simulink model "bh_explore_evassive_manoeuvre_automate"  (R2017b)
settings: Solver=ode45  StartTime=0.0  StopTime=20  FixedStep=0.001  RelTol=1e-5
undefined symbols (not defined in the file or in its folder): Peak_deg, Tw, vel_mpersec
libraries: simulink_extras x12, bh_cv_car_drc_library x1
settings Model: Creator=bhorton  LastModifiedBy=bhorton
settings SolverCC: ZeroCrossControl=EnableAll  ZeroCrossAlgorithm=Adaptive
settings DebuggingCC: SignalInfNanChecking=warning
settings ModelReferenceCC: ModelReferenceMinAlgLoopOccurrences=on

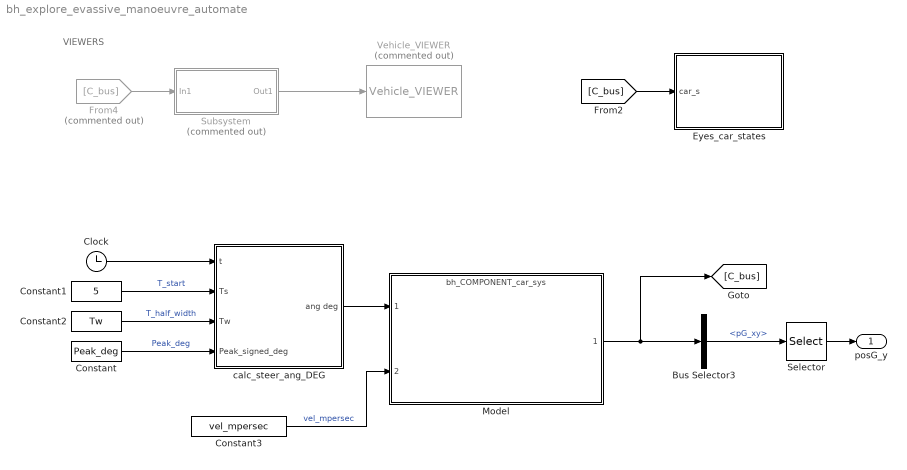
== system bh_explore_evassive_manoeuvre_automate ==
  note: VIEWERS
  Bus Selector3 : BusSelector  OutputSignals=states_G.pG_xy
  Clock : Clock
  Constant : Constant  Value=Peak_deg
  Constant1 : Constant  Value=5
  Constant2 : Constant  Value=Tw
  Constant3 : Constant  Value=vel_mpersec
  Eyes_car_states : Subsystem
  From4 : From  Commented=on  GotoTag=C_bus
  Model : ModelReference  ModelNameDialog=bh_COMPONENT_car_sys  SimulationMode=Normal  ModelReferenceVersion=1.261
  Selector : Selector  InputPortWidth=2  IndexOptions=Index vector (dialog)  Indices=2  OutputSizes=1
  Subsystem : Subsystem  Commented=on
  Vehicle_VIEWER : bh_cv_car_drc_library/CAR_things/Vehicle_VIEWER  Commented=on  wp_mat=[-1, -1; 2,2]  veh_ID_num=1  veh_init_xytheta=[0,0,0]  Ts=0.1
  calc_steer_ang_DEG : Subsystem
      mask Display: image(imread('evassive_PIC_01.JPG'))
  posG_y : Outport
  wires:
  [C_bus] -> Eyes_car_states/1(car_s)
  From4/1 -> Subsystem/1(In1)
  Subsystem/1(Out1) -> Vehicle_VIEWER/1
  Clock/1 -> calc_steer_ang_DEG/1(t)
  Constant/1 -> calc_steer_ang_DEG/4(Peak_signed_deg)  "Peak_deg"
  Constant1/1 -> calc_steer_ang_DEG/2(Ts)  "T_start"
  Constant2/1 -> calc_steer_ang_DEG/3(Tw)  "T_half_width"
  calc_steer_ang_DEG/1(ang deg) -> Model/1
  Constant3/1 -> Model/2  "vel_mpersec"
  Model/1 -> Bus Selector3/1, [C_bus]
  Bus Selector3/1 -> Selector/1  "<pG_xy>"
  Selector/1 -> posG_y/1

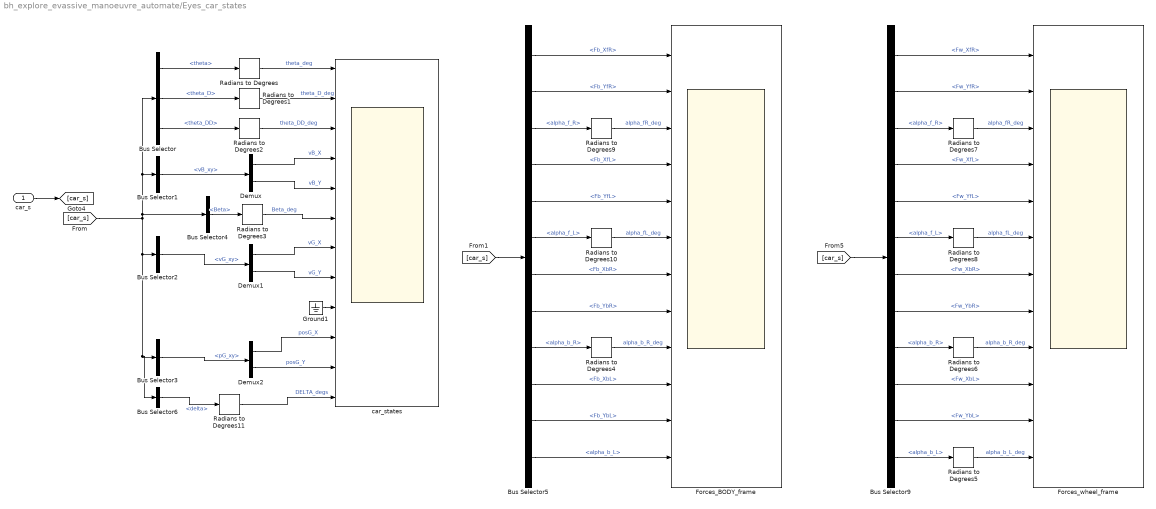
== system bh_explore_evassive_manoeuvre_automate/Eyes_car_states ==
  car_s : Inport
  Bus Selector : BusSelector  OutputSignals=states_B.theta,states_B.theta_D,states_B.theta_DD
  Bus Selector1 : BusSelector  OutputSignals=states_B.vB_xy
  Bus Selector2 : BusSelector  OutputSignals=states_G.vG_xy
  Bus Selector3 : BusSelector  OutputSignals=states_G.pG_xy
  Bus Selector4 : BusSelector  OutputSignals=states_B.Beta
  Bus Selector5 : BusSelector  OutputSignals=Force_BODY_frame.Fb_XfR,Force_BODY_frame.Fb_YfR,alpha.alpha_f_R,Force_BODY_frame.Fb_XfL,Force_BODY_frame.Fb_YfL,alpha.alpha_f_L,Force_BODY_frame.Fb_XbR,Force_BODY_frame.Fb_YbR,alpha.alpha_b_R,Force_BODY_frame.Fb_XbL,Force_BODY_frame.Fb_YbL,alpha.alpha_b_L
  Bus Selector6 : BusSelector  OutputSignals=wheel.delta
  Bus Selector9 : BusSelector  OutputSignals=Force_wheel_frame.Fw_XfR,Force_wheel_frame.Fw_YfR,alpha.alpha_f_R,Force_wheel_frame.Fw_XfL,Force_wheel_frame.Fw_YfL,alpha.alpha_f_L,Force_wheel_frame.Fw_XbR,Force_wheel_frame.Fw_YbR,alpha.alpha_b_R,Force_wheel_frame.Fw_XbL,Force_wheel_frame.Fw_YbL,alpha.alpha_b_L
  Demux : Demux  Outputs=2
  Demux1 : Demux  Outputs=2
  Demux2 : Demux  Outputs=2
  Forces_BODY_frame : Scope  NumInputPorts=12
  Forces_wheel_frame : Scope  NumInputPorts=12
  Ground1 : Ground
  Radians to Degrees{,1..11} (12 alike) : simulink_extras/Transformations/Radians to Degrees
  car_states : Scope  NumInputPorts=12
  wires:
  car_s/1 -> [car_s]
  [car_s] -> Bus Selector4/1, Bus Selector/1, Bus Selector1/1, Bus Selector6/1, Bus Selector3/1, Bus Selector2/1
  Bus Selector/1 -> Radians to Degrees/1  "<theta>"
  Bus Selector/2 -> Radians to Degrees1/1  "<theta_D>"
  Bus Selector/3 -> Radians to Degrees2/1  "<theta_DD>"
  Radians to Degrees/1 -> car_states/1  "theta_deg"
  Radians to Degrees1/1 -> car_states/2  "theta_D_deg"
  Radians to Degrees2/1 -> car_states/3  "theta_DD_deg"
  Bus Selector1/1 -> Demux/1  "<vB_xy>"
  Demux/1 -> car_states/4  "vB_X"
  Demux/2 -> car_states/5  "vB_Y"
  Radians to Degrees3/1 -> car_states/6  "Beta_deg"
  Bus Selector2/1 -> Demux1/1  "<vG_xy>"
  Demux1/1 -> car_states/7  "vG_X"
  Demux1/2 -> car_states/8  "vG_Y"
  Ground1/1 -> car_states/9
  Demux2/1 -> car_states/10  "posG_X"
  Demux2/2 -> car_states/11  "posG_Y"
  Bus Selector3/1 -> Demux2/1  "<pG_xy>"
  Radians to Degrees11/1 -> car_states/12  "DELTA_degs"
  Bus Selector4/1 -> Radians to Degrees3/1  "<Beta>"
  [car_s] -> Bus Selector9/1
  Bus Selector9/1 -> Forces_wheel_frame/1  "<Fw_XfR>"
  Bus Selector9/2 -> Forces_wheel_frame/2  "<Fw_YfR>"
  Bus Selector9/3 -> Radians to Degrees7/1  "<alpha_f_R>"
  Bus Selector9/4 -> Forces_wheel_frame/4  "<Fw_XfL>"
  Bus Selector9/5 -> Forces_wheel_frame/5  "<Fw_YfL>"
  Bus Selector9/6 -> Radians to Degrees8/1  "<alpha_f_L>"
  Bus Selector9/7 -> Forces_wheel_frame/7  "<Fw_XbR>"
  Bus Selector9/8 -> Forces_wheel_frame/8  "<Fw_YbR>"
  Bus Selector9/9 -> Radians to Degrees6/1  "<alpha_b_R>"
  Bus Selector9/10 -> Forces_wheel_frame/10  "<Fw_XbL>"
  Bus Selector9/11 -> Forces_wheel_frame/11  "<Fw_YbL>"
  Bus Selector9/12 -> Radians to Degrees5/1  "<alpha_b_L>"
  Radians to Degrees7/1 -> Forces_wheel_frame/3  "alpha_fR_deg"
  Radians to Degrees8/1 -> Forces_wheel_frame/6  "alpha_fL_deg"
  Radians to Degrees6/1 -> Forces_wheel_frame/9  "alpha_b_R_deg"
  Radians to Degrees5/1 -> Forces_wheel_frame/12  "alpha_b_L_deg"
  Radians to Degrees10/1 -> Forces_BODY_frame/6  "alpha_fL_deg"
  Radians to Degrees4/1 -> Forces_BODY_frame/9  "alpha_b_R_deg"
  Radians to Degrees9/1 -> Forces_BODY_frame/3  "alpha_fR_deg"
  Bus Selector5/9 -> Radians to Degrees4/1  "<alpha_b_R>"
  Bus Selector5/7 -> Forces_BODY_frame/7  "<Fb_XbR>"
  Bus Selector5/10 -> Forces_BODY_frame/10  "<Fb_XbL>"
  Bus Selector5/11 -> Forces_BODY_frame/11  "<Fb_YbL>"
  Bus Selector5/6 -> Radians to Degrees10/1  "<alpha_f_L>"
  Bus Selector5/5 -> Forces_BODY_frame/5  "<Fb_YfL>"
  Bus Selector5/4 -> Forces_BODY_frame/4  "<Fb_XfL>"
  Bus Selector5/8 -> Forces_BODY_frame/8  "<Fb_YbR>"
  Bus Selector5/2 -> Forces_BODY_frame/2  "<Fb_YfR>"
  [car_s] -> Bus Selector5/1
  Bus Selector5/3 -> Radians to Degrees9/1  "<alpha_f_R>"
  Bus Selector5/1 -> Forces_BODY_frame/1  "<Fb_XfR>"
  Bus Selector5/12 -> Forces_BODY_frame/12  "<alpha_b_L>"
  Bus Selector6/1 -> Radians to Degrees11/1  "<delta>"

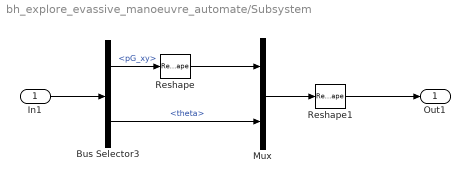
== system bh_explore_evassive_manoeuvre_automate/Subsystem ==
  In1 : Inport
  Bus Selector3 : BusSelector  OutputSignals=states_G.pG_xy,states_B.theta
  Mux : Mux  Inputs=2
  Reshape : Reshape  OutputDimensionality=Column vector (2-D)
  Reshape1 : Reshape  OutputDimensionality=Column vector (2-D)
  Out1 : Outport
  wires:
  In1/1 -> Bus Selector3/1
  Bus Selector3/1 -> Reshape/1  "<pG_xy>"
  Reshape/1 -> Mux/1
  Bus Selector3/2 -> Mux/2  "<theta>"
  Mux/1 -> Reshape1/1
  Reshape1/1 -> Out1/1

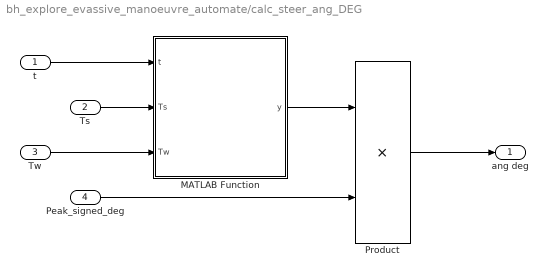
== system bh_explore_evassive_manoeuvre_automate/calc_steer_ang_DEG ==
  t : Inport
  Ts : Inport  Port=2
  Tw : Inport  Port=3
  Peak_signed_deg : Inport  Port=4
  MATLAB Function : MATLAB Function  TreatAsAtomicUnit=on
  Product : Product
  ang deg : Outport
  wires:
  t/1 -> MATLAB Function/1(t)
  Ts/1 -> MATLAB Function/2(Ts)
  Tw/1 -> MATLAB Function/3(Tw)
  MATLAB Function/1(y) -> Product/1
  Peak_signed_deg/1 -> Product/2
  Product/1 -> ang deg/1

== matlab function bh_explore_evassive_manoeuvre_automate/calc_steer_ang_DEG/MATLAB Function ==
  data: t input; y output; Ts input; Tw input
function y = fcn(t,Ts,Tw)

y = 0;

% first look for the out of bounds cases
if(  t <= Ts )
    return;
end

if( t >= (Ts + 2*Tw) )
    return;
end

%OK: if we're here then do your thing
m_climbing = 1/(Tw/2);
m_falling  = -1 * m_climbing;

if(  (t > Ts) && (t <= (Ts + Tw/2))  )
    % first CLIMBING zone
    t_star = t - Ts;
         y = t_star * m_climbing;
elseif(  (t > (Ts + Tw/2)) && (t <= (Ts + 3*Tw/2))   )
    % the FALLING zone
    t_star = t - (Ts + Tw/2);
         y = t_star * m_falling +  1;
else
    % the 2nd CLIMBING zone
    t_star = t - (Ts + 3*Tw/2);
         y = t_star * m_climbing -  1;
end
